simulink model "detumbling_sim_2020"  (R2024a)
settings: Solver=ode4  StartTime=0.0  StopTime=inf  FixedStep=0.001  RelTol=1e-3
settings Model: Creator=airmarshall  LastModifiedBy=maria
settings SolverCC: AlgebraicLoopSolver=TrustRegion
settings RTWCC: GPUComputeCapability=3.5  DLArmComputeVersion=19.05

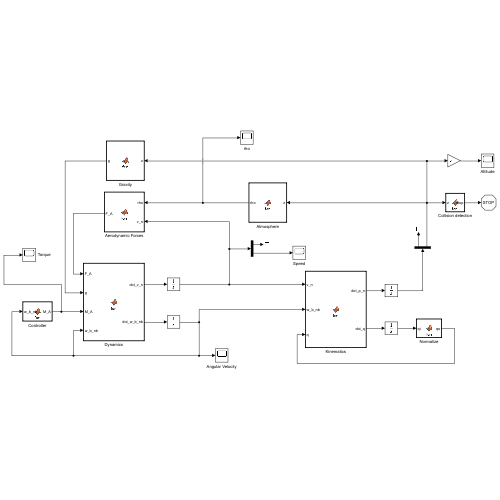
[thumbnail: Simulink's stored preview of the top-level diagram]
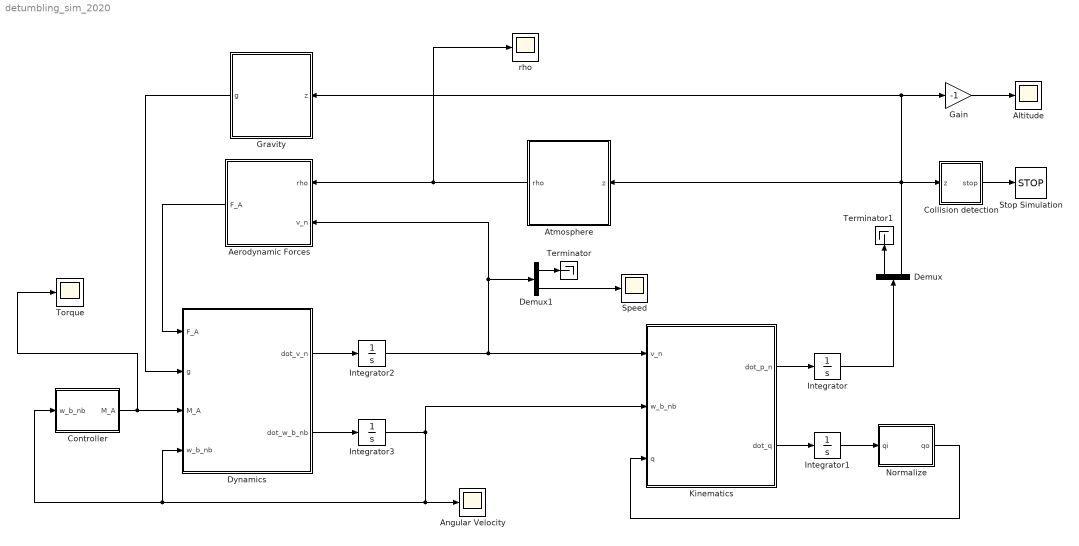
== system detumbling_sim_2020 ==
  Aerodynamic Forces : MATLAB Function  TreatAsAtomicUnit=on
  Altitude : Scope
  Angular Velocity : Scope
  Atmosphere : MATLAB Function  TreatAsAtomicUnit=on
  Collision detection : MATLAB Function  TreatAsAtomicUnit=on
  Controller : MATLAB Function  TreatAsAtomicUnit=on
  Demux : Demux  Outputs=[2;1]
  Demux1 : Demux  Outputs=[2;1]
  Dynamics : MATLAB Function  TreatAsAtomicUnit=on
  Gain : Gain  Gain=-1
  Gravity : MATLAB Function  TreatAsAtomicUnit=on
  Integrator : Integrator  InitialCondition=[0;0;-90000]
  Integrator1 : Integrator  InitialCondition=[1;0;0;0]
  Integrator2 : Integrator  InitialCondition=[0;0;-170*9.81]
  Integrator3 : Integrator  InitialCondition=12*pi*rand(3,1)/sqrt(3)
  Kinematics : MATLAB Function  TreatAsAtomicUnit=on
  Normalize : MATLAB Function  TreatAsAtomicUnit=on
  Speed : Scope
  Stop Simulation : Stop
  Terminator : Terminator
  Terminator1 : Terminator
  Torque : Scope
  rho : Scope
  wires:
  Integrator2/1 -> Demux1/1, Aerodynamic Forces/2(v_n), Kinematics/1(v_n)
  Integrator/1 -> Demux/1
  Dynamics/1(dot_v_n) -> Integrator2/1
  Integrator3/1 -> Kinematics/2(w_b_nb), Angular Velocity/1, Dynamics/4(w_b_nb), Controller/1(w_b_nb)
  Demux/2 -> Collision detection/1(z), Atmosphere/1(z), Gain/1, Gravity/1(z)
  Integrator1/1 -> Normalize/1(qi)
  Kinematics/2(dot_q) -> Integrator1/1
  Kinematics/1(dot_p_n) -> Integrator/1
  Aerodynamic Forces/1(F_A) -> Dynamics/1(F_A)
  Dynamics/2(dot_w_b_nb) -> Integrator3/1
  Controller/1(M_A) -> Torque/1, Dynamics/3(M_A)
  Collision detection/1(stop) -> Stop Simulation/1
  Normalize/1(qo) -> Kinematics/3(q)
  Gravity/1(g) -> Dynamics/2(g)
  Demux1/2 -> Speed/1
  Gain/1 -> Altitude/1
  Demux1/1 -> Terminator/1
  Demux/1 -> Terminator1/1
  Atmosphere/1(rho) -> rho/1, Aerodynamic Forces/1(rho)

== matlab function detumbling_sim_2020/Kinematics ==
  data: v_n input; w_b_nb input; dot_p_n output; q input; dot_q output
function [dot_p_n, dot_q] = fcn(v_n,w_b_nb,q)

dot_p_n = v_n;
dot_q = 1/2*qprod(q,v2q(w_b_nb));

end

function a = qprod(b,c)
    a = [b(1)*c(1)-dot(b(2:4),c(2:4));b(1)*c(2:4)+c(1)*b(2:4)+cross(b(2:4),c(2:4))];
end
function a = qconj(b)
    a = [b(1);-b(2:4)];
end
function a = q2v(b)
    a = b(2:4);
end
function a = v2q(b)
    a = [0;b(1:3)];
end
function a = qrot(b,c)
    a = q2v(qprod(b,qprod(v2q(c),qconj(b))));
end

== matlab function detumbling_sim_2020/Dynamics ==
  data: F_A input; g input; dot_v_n output; M_A input; w_b_nb input; dot_w_b_nb output
function [dot_v_n, dot_w_b_nb] = fcn(F_A,g, M_A, w_b_nb)
m = 2.66;
Jxx = 1/12*m*(0.1^2+0.2^2);
Jyy = 1/12*m*(0.2^2+0.1^2);
Jzz = 1/12*m*(0.1^2+0.1^2);
J = [Jxx 0 0;
     0 Jyy 0;
     0 0 Jzz];


F = [0;0;m*g]+F_A;
dot_v_n = 1/m*F;
dot_w_b_nb = J\(M_A - cross(w_b_nb, J*w_b_nb));

end

function a = qprod(b,c)
    a = [b(1)*c(1)-dot(b(2:4),c(2:4));b(1)*c(2:4)+c(1)*b(2:4)+cross(b(2:4),c(2:4))];
end
function a = qconj(b)
    a = [b(1);-b(2:4)];
end
function a = q2v(b)
    a = b(2:4);
end
function a = v2q(b)
    a = [0;b(1:3)];
end
function a = qrot(b,c)
    a = q2v(qprod(b,qprod(v2q(c),qconj(b))));
end

== matlab function detumbling_sim_2020/Controller ==
  data: w_b_nb input; M_A output
function M_A = fcn(w_b_nb)
%t_max = 1.6769e-04; %Reaction wheel
%t_max = 5e-04; %Ideal max torque?
t_max = 450*10-6; %Magnetic torquer (maximum)
k_w = 0.01;
M_A = -k_w*w_b_nb;
if norm(M_A) > t_max
    M_A = M_A/norm(M_A)*t_max;
end
end

== matlab function detumbling_sim_2020/Aerodynamic Forces ==
  data: rho input; v_n input; F_A output
function F_A  = fcn(rho,v_n)

S = 0.1^2;
V = norm(v_n);

C_D = 0.9;

q_bar = 1/2*rho*V^2;
F_A = [0;0;-q_bar*S*C_D];
end

== matlab function detumbling_sim_2020/Collision detection ==
  data: z input; stop output
function stop  = fcn(z)
if z > 0
    stop = 1;
else
    stop = 0;
end
end

== matlab function detumbling_sim_2020/Normalize ==
  data: qi input; qo output
function qo  = fcn(qi)
qo = qi/norm(qi);
end

== matlab function detumbling_sim_2020/Gravity ==
  data: z input; g output
function g  = fcn(z)
if z > 0
    g = 9.81;
else
r = abs(z) + 6371000;
g = 6.67e-11*5.97e24/r^2;
end
end

== matlab function detumbling_sim_2020/Atmosphere ==
  data: z input; rho output
function rho  = fcn(z)
h = abs(z);
if h > 25000
    T = -131.21+0.00299*h;
    p = 2.488*((T+273.1)/216.6)^(-11.388);
elseif h > 11000
    T = -56.46;
    p = 22.65*exp(1.73-0.000157*h);
else
    T = 15.04 - 0.00649*h;
    p = 101.29*((T+273.1)/288.08)^(5.256);
end
rho = p/(0.2869*(T+273.1));
end
